simulink model "ProjectCubeSat"  (R2022a)
settings: Solver=VariableStepAuto  StartTime=0.0  StopTime=10.0  RelTol=1e-3
settings Model: Creator=LabPC  LastModifiedBy=LabPC

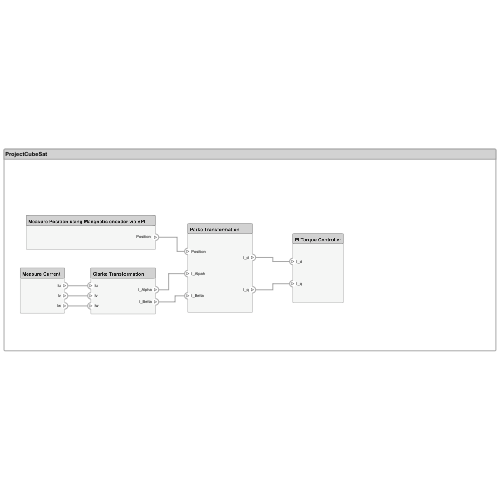
[thumbnail: Simulink's stored preview of the top-level diagram]
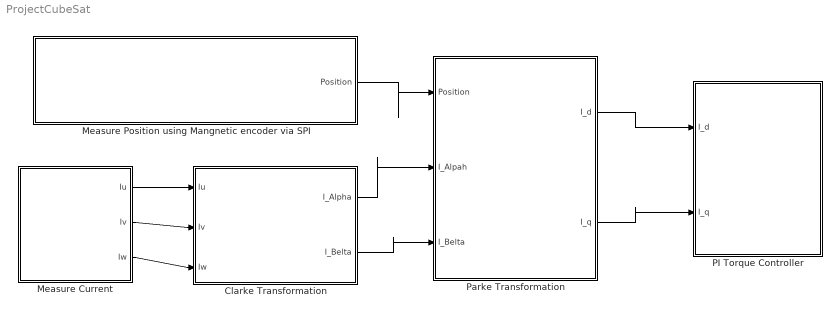
== system ProjectCubeSat ==
  "Clarke Transformation " : Subsystem
      settings: PortSchema="{\"entries\":[{\"content\":{\"headerSize\":26,\"margin\":15,\"minimumSpacing\":25,\"sides\":[{\"content\":{\"connectorIds\":[\"In1\",\"In2\",\"In3\"]},\"type\":\"ConnectorPlacement.EquallySpacedRectSide\",\"uuid\":\"686dc177-8139-4c04-a071-3511fd51c951\"},{\"content\":{\"connectorIds\":[\"Out1\",\"Out2\"],\"side\":\"RIGHT\"},\"type\":\"ConnectorPlacement.EquallySpacedRectSide\",\"uuid\":\"82c189bc-0b10-4c4e-a597-02026ca398d9\"},{\"content\":{\"connectorIds\":[],\"side\":\"TOP\"},\"type\":\"ConnectorPlacement.EquallySpacedRectSide\",\"uuid\":\"e730ed7c-55f1-4c3f-b42b-ff11075c27a3\"}]},\"type\":\"ConnectorPlacement.EquallySpacedConnector\",\"uuid\":\"9fcd88da-1b45-4ca2-9454-28a8a7109954\"}],\"packageUris\":[\"http://schema.mathworks.com/mf0/Connector/R2020b\"],\"version\":\"1.0\"}"
  "Measure Current " : Subsystem
      settings: PortSchema="{\"entries\":[{\"content\":{\"headerSize\":26,\"margin\":15,\"minimumSpacing\":25,\"sides\":[{\"content\":{\"connectorIds\":[]},\"type\":\"ConnectorPlacement.EquallySpacedRectSide\",\"uuid\":\"686dc177-8139-4c04-a071-3511fd51c951\"},{\"content\":{\"connectorIds\":[\"Out1\",\"Out2\",\"Out3\"],\"side\":\"RIGHT\"},\"type\":\"ConnectorPlacement.EquallySpacedRectSide\",\"uuid\":\"82c189bc-0b10-4c4e-a597-02026ca398d9\"},{\"content\":{\"connectorIds\":[],\"side\":\"TOP\"},\"type\":\"ConnectorPlacement.EquallySpacedRectSide\",\"uuid\":\"e730ed7c-55f1-4c3f-b42b-ff11075c27a3\"}]},\"type\":\"ConnectorPlacement.EquallySpacedConnector\",\"uuid\":\"9fcd88da-1b45-4ca2-9454-28a8a7109954\"}],\"packageUris\":[\"http://schema.mathworks.com/mf0/Connector/R2020b\"],\"version\":\"1.0\"}"
  Measure Position using Mangnetic encoder via SPI : Subsystem
      settings: PortSchema="{\"entries\":[{\"content\":{\"headerSize\":26,\"margin\":15,\"minimumSpacing\":25,\"sides\":[{\"content\":{\"connectorIds\":[]},\"type\":\"ConnectorPlacement.EquallySpacedRectSide\",\"uuid\":\"686dc177-8139-4c04-a071-3511fd51c951\"},{\"content\":{\"connectorIds\":[\"Out1\"],\"side\":\"RIGHT\"},\"type\":\"ConnectorPlacement.EquallySpacedRectSide\",\"uuid\":\"82c189bc-0b10-4c4e-a597-02026ca398d9\"},{\"content\":{\"connectorIds\":[],\"side\":\"TOP\"},\"type\":\"ConnectorPlacement.EquallySpacedRectSide\",\"uuid\":\"e730ed7c-55f1-4c3f-b42b-ff11075c27a3\"}]},\"type\":\"ConnectorPlacement.EquallySpacedConnector\",\"uuid\":\"9fcd88da-1b45-4ca2-9454-28a8a7109954\"}],\"packageUris\":[\"http://schema.mathworks.com/mf0/Connector/R2020b\"],\"version\":\"1.0\"}"
  PI Torque Controller : Subsystem
      settings: PortSchema="{\"entries\":[{\"content\":{\"headerSize\":26,\"margin\":15,\"minimumSpacing\":25,\"sides\":[{\"content\":{\"connectorIds\":[\"In2\",\"In1\"]},\"type\":\"ConnectorPlacement.EquallySpacedRectSide\",\"uuid\":\"686dc177-8139-4c04-a071-3511fd51c951\"},{\"content\":{\"connectorIds\":[],\"side\":\"RIGHT\"},\"type\":\"ConnectorPlacement.EquallySpacedRectSide\",\"uuid\":\"82c189bc-0b10-4c4e-a597-02026ca398d9\"},{\"content\":{\"connectorIds\":[],\"side\":\"TOP\"},\"type\":\"ConnectorPlacement.EquallySpacedRectSide\",\"uuid\":\"e730ed7c-55f1-4c3f-b42b-ff11075c27a3\"},{\"content\":{\"connectorIds\":[],\"side\":\"BOTTOM\"},\"type\":\"ConnectorPlacement.EquallySpacedRectSide\",\"uuid\":\"ef60c478-6361-474b-b12d-24dfb02c2ddd\"}]},\"type\":\"ConnectorPlacement.EquallySpacedConnector\",\"uuid\":\"9fcd88da-1b45-4ca2-9454-28a8a7109954\"}],\"packageUris\":[\"http://schema.mathworks.com/mf0/Connector/R2020b\"],\"version\":\"1.0\"}"
  "Parke Transformation " : Subsystem
      settings: PortSchema="{\"entries\":[{\"content\":{\"headerSize\":26,\"margin\":15,\"minimumSpacing\":25,\"sides\":[{\"content\":{\"connectorIds\":[\"In1\",\"In2\",\"In3\"]},\"type\":\"ConnectorPlacement.EquallySpacedRectSide\",\"uuid\":\"686dc177-8139-4c04-a071-3511fd51c951\"},{\"content\":{\"connectorIds\":[\"Out1\",\"Out2\"],\"side\":\"RIGHT\"},\"type\":\"ConnectorPlacement.EquallySpacedRectSide\",\"uuid\":\"82c189bc-0b10-4c4e-a597-02026ca398d9\"},{\"content\":{\"connectorIds\":[],\"side\":\"TOP\"},\"type\":\"ConnectorPlacement.EquallySpacedRectSide\",\"uuid\":\"e730ed7c-55f1-4c3f-b42b-ff11075c27a3\"}]},\"type\":\"ConnectorPlacement.EquallySpacedConnector\",\"uuid\":\"9fcd88da-1b45-4ca2-9454-28a8a7109954\"}],\"packageUris\":[\"http://schema.mathworks.com/mf0/Connector/R2020b\"],\"version\":\"1.0\"}"
  wires:
  "Measure Current "/2(Iv) -> "Clarke Transformation "/2(Iv)
  "Measure Current "/3(Iw) -> "Clarke Transformation "/3(Iw)
  "Measure Current "/1(Iu) -> "Clarke Transformation "/1(Iu)
  "Clarke Transformation "/1(I_Alpha) -> "Parke Transformation "/2(I_Alpah)
  "Clarke Transformation "/2(I_Belta) -> "Parke Transformation "/3(I_Belta)
  Measure Position using Mangnetic encoder via SPI/1("Position ") -> "Parke Transformation "/1("Position ")
  "Parke Transformation "/1(I_d) -> PI Torque Controller/2(I_d)
  "Parke Transformation "/2(I_q) -> PI Torque Controller/1(I_q)

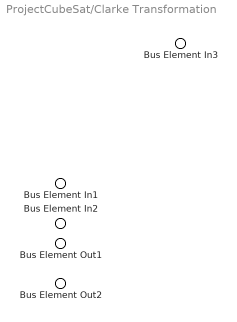
== system ProjectCubeSat/Clarke Transformation  ==
  Bus Element In3 : Inport  PortName=Iu
  Bus Element In1 : Inport  Port=2  PortName=Iv
  Bus Element In2 : Inport  Port=3  PortName=Iw
  Bus Element Out1 : Outport  PortName=I_Alpha
  Bus Element Out2 : Outport  Port=2  PortName=I_Belta

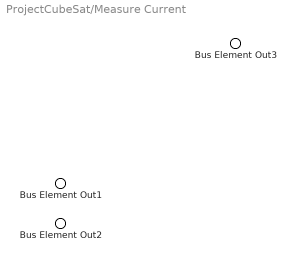
== system ProjectCubeSat/Measure Current  ==
  Bus Element Out3 : Outport  PortName=Iu
  Bus Element Out1 : Outport  Port=2  PortName=Iv
  Bus Element Out2 : Outport  Port=3  PortName=Iw

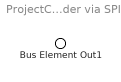
== system ProjectCubeSat/Measure Position using Mangnetic encoder via SPI ==
  Bus Element Out1 : Outport  PortName=Position

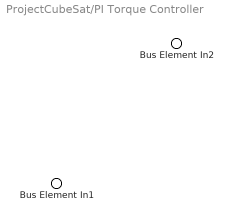
== system ProjectCubeSat/PI Torque Controller ==
  Bus Element In2 : Inport  PortName=I_q
  Bus Element In1 : Inport  Port=2  PortName=I_d

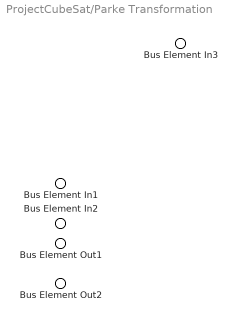
== system ProjectCubeSat/Parke Transformation  ==
  Bus Element In3 : Inport  PortName=Position
  Bus Element In1 : Inport  Port=2  PortName=I_Alpah
  Bus Element In2 : Inport  Port=3  PortName=I_Belta
  Bus Element Out1 : Outport  PortName=I_d
  Bus Element Out2 : Outport  Port=2  PortName=I_q
